simulink model "frequency_hopping"  (R2018b)
settings: Solver=FixedStepDiscrete  StartTime=0.0  StopTime=900*1  RelTol=1e-3
libraries: hdlsllib x4, simulink x2
settings Model: DataTypeOverride=Off  Creator=tcollins  LastModifiedBy=tcollins
settings DataIOCC: LimitDataPoints=on  SaveOutput=off  SaveTime=off
settings OptimizationCC: BlockReduction=off  ConditionallyExecuteInputs=off  DefaultParameterBehavior=Inlined  LifeSpan=inf
settings DebuggingCC: AlgebraicLoopMsg=error  SingleTaskRateTransMsg=error  AllowSymbolicDim=off  StrictBusMsg=ErrorOnBusTreatedAsVector  SFUnexpectedBacktrackingDiag=warning  SFNoUnconditionalDefaultTransitionDiag=warning  SFExecutionAtInitializationDiag=none
settings HardwareCC: ProdBitPerPointer=32  ProdBitPerSizeT=32  ProdBitPerPtrDiffT=32  ProdLargestAtomicFloat=None  ProdIntDivRoundTo=Undefined  ProdEndianess=Unspecified  ProdWordSize=32  ProdHWDeviceType=ASIC/FPGA->ASIC/FPGA  ProdEqTarget=off
settings SFSimCC: SimUseLocalCustomCode=off
settings RTWCC: RTWUseLocalCustomCode=off
settings CodeAppCC: StateflowObjectComments=on
settings GRTTargetCC: TargetLangStandard=C89/C90 (ANSI)  GeneratePreprocessorConditionals=Disable all
settings ConfigComp: CovScope=ReferencedModels  CovMetricSettings=dw  CovHtmlReporting=on  CovSaveCumulativeToWorkspaceVar=on  CovSaveSingleToWorkspaceVar=on  CovExternalEMLEnable=off  CovSFcnEnable=off

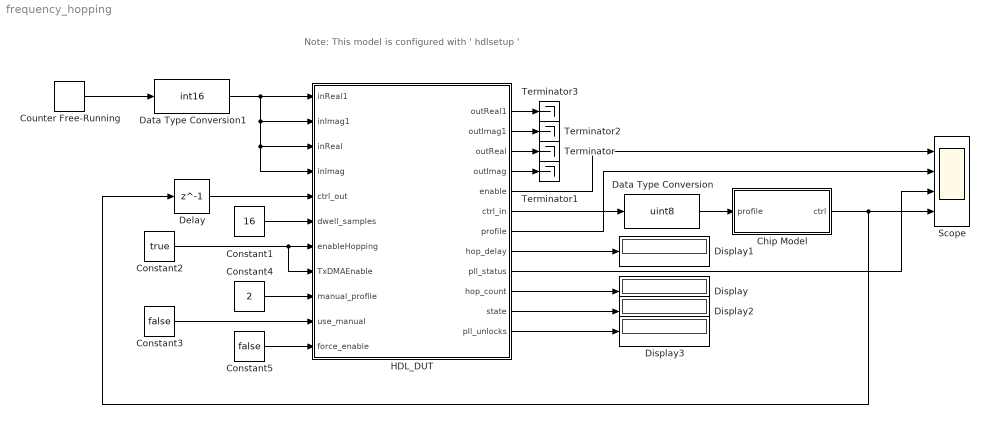
== system frequency_hopping ==
  note: Note: This model is configured with ' hdlsetup '
  Chip Model : MATLAB Function  TreatAsAtomicUnit=on
  Constant1 : Constant  Value=16  OutDataTypeStr=fixdt(1,16,0)  SampleTime=-1
  Constant2 : Constant  Value=true  OutDataTypeStr=boolean  SampleTime=-1
  Constant3 : Constant  Value=false  OutDataTypeStr=boolean  SampleTime=-1
  Constant4 : Constant  Value=2  OutDataTypeStr=uint32  SampleTime=-1
  Constant5 : Constant  Value=false  OutDataTypeStr=boolean  SampleTime=-1
  Counter Free-Running : simulink/Sources/Counter Free-Running  NumBits=10  tsamp=1
  Data Type Conversion : DataTypeConversion  OutDataTypeStr=uint8
  Data Type Conversion1 : DataTypeConversion  OutDataTypeStr=int16
  Delay : Delay  DelayLength=1
  Display{,1..3} (4 alike) : Display
  HDL_DUT : Subsystem  TreatAsAtomicUnit=on
  Scope : Scope  NumInputPorts=4
  Terminator{,1..3} (4 alike) : Terminator
  wires:
  Counter Free-Running/1 -> Data Type Conversion1/1
  Delay/1 -> HDL_DUT/5(ctrl_out)
  Constant1/1 -> HDL_DUT/6(dwell_samples)
  Chip Model/1(ctrl) -> Scope/4, Delay/1
  HDL_DUT/6(ctrl_in) -> Data Type Conversion/1
  Data Type Conversion/1 -> Chip Model/1(profile)
  Data Type Conversion1/1 -> HDL_DUT/4(inImag), HDL_DUT/3(inReal), HDL_DUT/2(inImag1), HDL_DUT/1(inReal1)
  HDL_DUT/3(outReal) -> Terminator/1
  HDL_DUT/4(outImag) -> Terminator1/1
  HDL_DUT/10(hop_count) -> Display/1
  HDL_DUT/8(hop_delay) -> Display1/1
  Constant2/1 -> HDL_DUT/8(TxDMAEnable), HDL_DUT/7(enableHopping)
  HDL_DUT/1(outReal1) -> Terminator3/1
  HDL_DUT/2(outImag1) -> Terminator2/1
  HDL_DUT/11(state) -> Display2/1
  HDL_DUT/12(pll_unlocks) -> Display3/1
  Constant3/1 -> HDL_DUT/10(use_manual)
  Constant4/1 -> HDL_DUT/9(manual_profile)
  HDL_DUT/9(pll_status) -> Scope/3
  HDL_DUT/5(enable) -> Scope/1
  HDL_DUT/7(profile) -> Scope/2
  Constant5/1 -> HDL_DUT/11(force_enable)

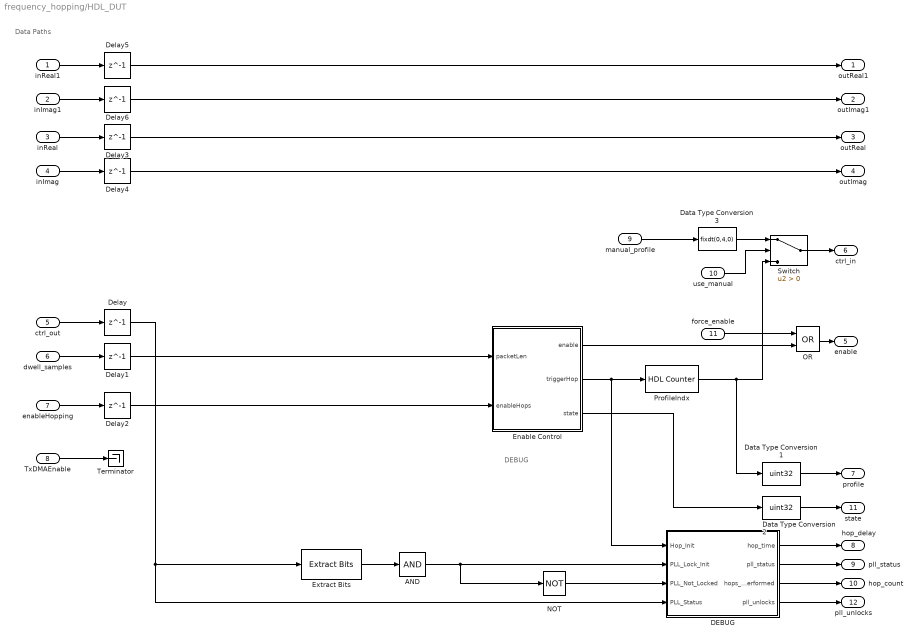
== system frequency_hopping/HDL_DUT ==
  note: DEBUG
  note: Data Paths
  inReal1 : Inport
  inImag1 : Inport  Port=2
  inReal : Inport  Port=3
  inImag : Inport  Port=4
  ctrl_out : Inport  Port=5
  dwell_samples : Inport  Port=6
  enableHopping : Inport  Port=7  OutDataTypeStr=boolean
  TxDMAEnable : Inport  Port=8  OutDataTypeStr=boolean
  manual_profile : Inport  Port=9  OutDataTypeStr=uint32
  use_manual : Inport  Port=10  OutDataTypeStr=boolean
  force_enable : Inport  Port=11  OutDataTypeStr=boolean
  AND : Logic  Inputs=1  AllPortsSameDT=off  OutDataTypeStr=boolean
  DEBUG : Subsystem
  Data Type Conversion1 : DataTypeConversion  OutDataTypeStr=uint32
  Data Type Conversion2 : DataTypeConversion  OutDataTypeStr=uint32
  Data Type Conversion3 : DataTypeConversion  OutDataTypeStr=fixdt(0,4,0)  SaturateOnIntegerOverflow=on
  Delay{,1..6} (7 alike) : Delay  DelayLength=1
  Enable Control : MATLAB Function  TreatAsAtomicUnit=on
  Extract Bits : simulink/Logic and Bit Operations/Extract Bits  bitsToExtract=Range of bits  numBits=8  bitIdxRange=[5 7]  outScalingMode=Preserve fixed-point scaling
      settings: SourceProductName=Simulink
  NOT : Logic  Operator=NOT  IconShape=distinctive  AllPortsSameDT=off  OutDataTypeStr=boolean
  OR : Logic  Operator=OR  AllPortsSameDT=off  OutDataTypeStr=boolean
  ProfileIndx : hdlsllib/Sources/HDL Counter  CountType=Count limited  CountInit=0  CountStep=2  CountMax=15  CountFromType=Initial value  CountFrom=0  CountResetPort=off  CountLoadPort=off  CountEnbPort=on  CountDirPort=off  CountDataType=Unsigned  CountWordLen=4  CountFracLen=0  CountSampTime=1
      settings: SourceProductBaseCode=HD
  Switch : Switch  Criteria=u2 > Threshold
  Terminator : Terminator
  outReal1 : Outport
  outImag1 : Outport  Port=2
  outReal : Outport  Port=3
  outImag : Outport  Port=4
  enable : Outport  Port=5
  ctrl_in : Outport  Port=6
  profile : Outport  Port=7
  hop_delay : Outport  Port=8
  pll_status : Outport  Port=9
  hop_count : Outport  Port=10
  state : Outport  Port=11
  pll_unlocks : Outport  Port=12
  wires:
  dwell_samples/1 -> Delay1/1
  ctrl_out/1 -> Delay/1
  Delay/1 -> Extract Bits/1, DEBUG/4(PLL_Status)
  Delay1/1 -> Enable Control/1(packetLen)
  Enable Control/2(triggerHop) -> DEBUG/1(Hop_Init), ProfileIndx/1
  inReal/1 -> Delay3/1
  inImag/1 -> Delay4/1
  Delay3/1 -> outReal/1
  Delay4/1 -> outImag/1
  DEBUG/1(hop_time) -> hop_delay/1
  DEBUG/2(pll_status) -> pll_status/1
  DEBUG/3(hops_performed) -> hop_count/1
  Data Type Conversion1/1 -> profile/1
  enableHopping/1 -> Delay2/1
  Delay2/1 -> Enable Control/2(enableHops)
  TxDMAEnable/1 -> Terminator/1
  Delay6/1 -> outImag1/1
  Delay5/1 -> outReal1/1
  inImag1/1 -> Delay6/1
  inReal1/1 -> Delay5/1
  ProfileIndx/1 -> Switch/3, Data Type Conversion1/1
  Data Type Conversion2/1 -> state/1
  Enable Control/3(state) -> Data Type Conversion2/1
  DEBUG/4(pll_unlocks) -> pll_unlocks/1
  manual_profile/1 -> Data Type Conversion3/1
  Switch/1 -> ctrl_in/1
  use_manual/1 -> Switch/2
  Data Type Conversion3/1 -> Switch/1
  Enable Control/1(enable) -> OR/2
  force_enable/1 -> OR/1
  OR/1 -> enable/1
  NOT/1 -> DEBUG/3(PLL_Not_Locked)
  Extract Bits/1 -> AND/1
  AND/1 -> DEBUG/2(PLL_Lock_Init), NOT/1

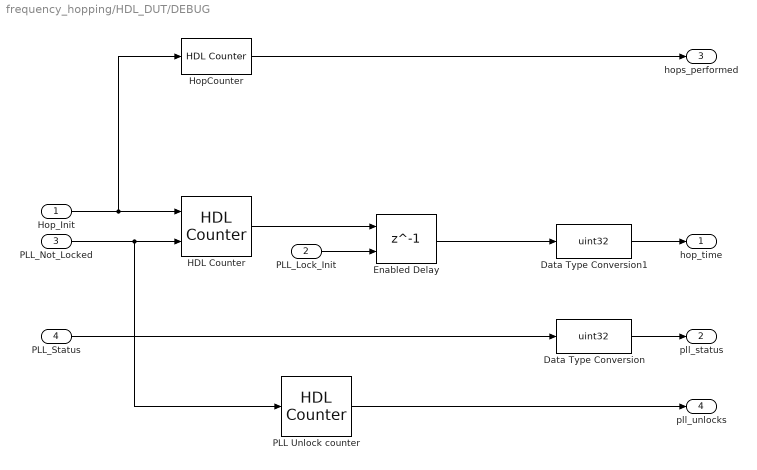
== system frequency_hopping/HDL_DUT/DEBUG ==
  Hop_Init : Inport
  PLL_Lock_Init : Inport  Port=2
  PLL_Not_Locked : Inport  Port=3
  PLL_Status : Inport  Port=4
  Data Type Conversion : DataTypeConversion  OutDataTypeStr=uint32
  Data Type Conversion1 : DataTypeConversion  OutDataTypeStr=uint32
  Enabled Delay : Delay  DelayLength=1  ShowEnablePort=on
      settings: InputPortMap=u0,e6
  HDL Counter : hdlsllib/Sources/HDL Counter  CountType=Count limited  CountInit=0  CountStep=1  CountMax=2^15  CountFromType=Initial value  CountFrom=0  CountResetPort=on  CountLoadPort=off  CountEnbPort=on  CountDirPort=off  CountDataType=Unsigned  CountWordLen=16  CountFracLen=0  CountSampTime=1
      settings: SourceProductBaseCode=HD
  HopCounter : hdlsllib/Sources/HDL Counter  CountType=Count limited  CountInit=0  CountStep=1  CountMax=2^31  CountFromType=Initial value  CountFrom=0  CountResetPort=off  CountLoadPort=off  CountEnbPort=on  CountDirPort=off  CountDataType=Unsigned  CountWordLen=32  CountFracLen=0  CountSampTime=1
      settings: SourceProductBaseCode=HD
  PLL Unlock counter : hdlsllib/Sources/HDL Counter  CountType=Count limited  CountInit=0  CountStep=1  CountMax=2^15  CountFromType=Initial value  CountFrom=0  CountResetPort=off  CountLoadPort=off  CountEnbPort=on  CountDirPort=off  CountDataType=Unsigned  CountWordLen=32  CountFracLen=0  CountSampTime=1
      settings: SourceProductBaseCode=HD
  hop_time : Outport
  pll_status : Outport  Port=2
  hops_performed : Outport  Port=3
  pll_unlocks : Outport  Port=4
  wires:
  PLL_Lock_Init/1 -> Enabled Delay/2
  HDL Counter/1 -> Enabled Delay/1
  Hop_Init/1 -> HopCounter/1, HDL Counter/1
  Enabled Delay/1 -> Data Type Conversion1/1
  PLL_Status/1 -> Data Type Conversion/1
  Data Type Conversion1/1 -> hop_time/1
  Data Type Conversion/1 -> pll_status/1
  HopCounter/1 -> hops_performed/1
  PLL_Not_Locked/1 -> PLL Unlock counter/1, HDL Counter/2
  PLL Unlock counter/1 -> pll_unlocks/1

== matlab function frequency_hopping/HDL_DUT/Enable Control ==
  data: enable output; packetLen input; triggerHop output; enableHops input; state output
function [enable,triggerHop,state] = fcn(packetLen, enableHops)


persistent counter counterLock

if isempty(counter)
    counter = uint16(0);
    counterLock = uint16(0);
end

waitSamples = 20;

% Start hop convergence wait
if counter == uint16(0) && enableHops
    counter = uint16(packetLen);
    counterLock = uint16(waitSamples);
    triggerHop = false;
    enable = false;
    state = uint8(0);
% Cycle through PLL lock period
elseif counterLock > uint16(1)
    counterLock = counterLock - uint16(1);
    triggerHop = false;
    enable = false;
    state = uint8(1);
% Cycle through dwell period
elseif counter > uint16(1)
    counter = counter - uint16(1);
    triggerHop = false;
    enable = true;
    state = uint8(2);
% Trigger hop at end of dwell
elseif counter == uint16(1) && enableHops
    counter = counter - uint16(1);
    triggerHop = true;
    enable = true;
    state = uint8(3);
% Waiting for enable hop external signal
else
    triggerHop = false;
    enable = false;
    state = uint8(4);
end

== matlab function frequency_hopping/Chip Model ==
  data: ctrl output; profile input
function ctrl = fcn(profile)

persistent lastProfile counter

if isempty(lastProfile)
    lastProfile = uint8(0);
    counter = 0;
end


if counter>=0
    counter = counter - 1;
    ctrl = uint8(0);
else
    ctrl = uint8(2^8-1);
end

if profile~=lastProfile
    lastProfile = profile;
    ctrl = uint8(0);
    counter = 32;
end
